simulink library "Floorheating_TABS"  (R2018b)
settings: Solver=ode45  StartTime=0.0  StopTime=10.0  RelTol=1e-3  EnableMultiTasking=on
settings Model: Creator=lena.frank  LastModifiedBy=drhf
settings DataIOCC: LimitDataPoints=on  SaveFormat=Array  SignalLoggingSaveFormat=ModelDataLogs
settings OptimizationCC: ExpressionDepthLimit=2147483647  LifeSpan=inf
settings DebuggingCC: UnderspecifiedInitializationDetection=Classic  MergeDetectMultiDrivingBlocksExec=none  SolverPrmCheckMsg=warning  FcnCallInpInsideContextMsg=warning  StateNameClashWarn=warning  SFUnexpectedBacktrackingDiag=warning  SFNoUnconditionalDefaultTransitionDiag=warning  SFExecutionAtInitializationDiag=none
settings HardwareCC: ProdBitPerPointer=32  ProdBitPerSizeT=32  ProdBitPerPtrDiffT=32  ProdLargestAtomicFloat=None  ProdIntDivRoundTo=Undefined  ProdEndianess=Unspecified  ProdWordSize=32  ProdHWDeviceType=32-bit Generic
settings ModelReferenceCC: PropagateSignalLabelsOutOfModel=off
settings SFSimCC: SimUseLocalCustomCode=off
settings RTWCC: RTWUseLocalCustomCode=off
settings CodeAppCC: StateflowObjectComments=on
settings GRTTargetCC: TargetLangStandard=C89/C90 (ANSI)  GeneratePreprocessorConditionals=Disable all  CombineOutputUpdateFcns=off  GRTInterface=on
settings ConfigComp: CovMetricSettings=dw  CovHtmlReporting=on  CovSaveCumulativeToWorkspaceVar=on  CovSaveSingleToWorkspaceVar=on  CovExternalEMLEnable=off

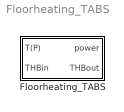
== system Floorheating_TABS ==
  Floorheating_TABS : Subsystem  mask(FBH-TABS){d=0.08, d1=0.04, d_pipe=0.016, dr=0.002, dx=0.1, l=700, lambda_r=0.35, lambda_b=1.4}
      mask prompts: d "thickness of active layer [m]"; d1 "depth of pipes in active layer [m]"; d_pipe "outer diameter of pipes [m]"; dr "wall thickness of pipe [m]"; dx "distance between center of pipes [m]"; l "length of pipe [m]"; lambda_r "conductivity of pipe [W/(m*K)]"; lambda_b "conductivity of layer material [W/(m*K)]"
      mask help:
      | calculates the heating/cooling power from pipes
      | in a floor heating system or a thermally active building component
      | to the active layer in the building element (wall, floor, ceiling)
      | according to the model of M.Koschenz & B.Lehmann, EMPA-CH, 2000
      mask Help: web(fullfile(path_carnot('help'),'FHB_TABS.html'),'-helpbrowser')

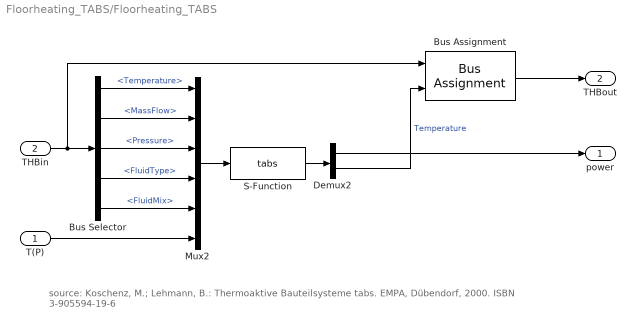
== system Floorheating_TABS/Floorheating_TABS ==
  note: source: Koschenz, M.; Lehmann, B.: Thermoaktive Bauteilsysteme tabs. EMPA, Dübendorf, 2000. ISBN 3-905594-19-6
  T(P) : Inport
  THBin : Inport  Port=2
  Bus Assignment : BusAssignment  AssignedSignals=Temperature
  Bus Selector : BusSelector  OutputSignals=Temperature,MassFlow,Pressure,FluidType,FluidMix
  Demux2 : Demux  Outputs=2
  Mux2 : Mux  Inputs=6
  S-Function : S-Function  FunctionName=tabs  Parameters=d d1 d_pipe dr dx l lambda_r lambda_b  SFunctionDeploymentMode=off  EnableBusSupport=off
  power : Outport
  THBout : Outport  Port=2  InitialOutput=0
  wires:
  Bus Assignment/1 -> THBout/1
  Demux2/1 -> power/1
  Demux2/2 -> Bus Assignment/2  "Temperature"
  S-Function/1 -> Demux2/1
  Mux2/1 -> S-Function/1
  Bus Selector/1 -> Mux2/1  "<Temperature>"
  Bus Selector/5 -> Mux2/5  "<FluidMix>"
  Bus Selector/2 -> Mux2/2  "<MassFlow>"
  Bus Selector/3 -> Mux2/3  "<Pressure>"
  Bus Selector/4 -> Mux2/4  "<FluidType>"
  THBin/1 -> Bus Selector/1, Bus Assignment/1
  T(P)/1 -> Mux2/6
